simulink model "KalmanFilter_test"  (R2019a)
settings: Solver=FixedStepAuto  StartTime=0.0  StopTime=15  RelTol=1e-3  EnableMultiTasking=on
undefined symbols (not defined in the file): A, B, Ck, Discrete, Dk, i0, R, Time, Ts, u0, y0
libraries: MagnetoLibrary x3, ctrlSharedLib x1
settings Model: SimulationMode=external  ExtModeTrigDuration=2  Creator=jakub  LastModifiedBy=jakub
settings OptimizationCC: EnhancedBackFolding=on  PassReuseOutputArgsAs=Individual arguments  MaxStackSize=64  OptimizeBlockOrder=speed  DifferentSizesBufferReuse=on  OptimizationCustomize=off
settings DebuggingCC: ParameterTunabilityLossMsg=error
settings HardwareCC: ProdBitPerPointer=32  ProdBitPerSizeT=32  ProdBitPerPtrDiffT=32  ProdLargestAtomicInteger=Long  ProdLargestAtomicFloat=Double  ProdWordSize=32  ProdHWDeviceType=ARM Compatible->ARM Cortex
settings SFSimCC: MATLABDynamicMemAlloc=off
settings RTWCC: SystemTargetFile=ert.tlc  HardwareBoard=Arduino Due  TLCOptions=-aInlineSetEventsForThisBaseRateFcn=TLC_FALSE -aSuppressMultiTaskScheduler=TLC_FALSE -aRateBasedStepFcn=1  TemplateMakefile=ert_default_tmf  GenerateReport=on  Toolchain=Arduino ARM  BuildConfiguration=Faster Runs  IncludeHyperlinkInReport=on  LaunchReport=on  GenerateTraceInfo=on  GenerateTraceReport=on  GenerateTraceReportSl=on  GenerateTraceReportSf=on  GenerateTraceReportEml=on
settings CodeAppCC: ForceParamTrailComments=on  IgnoreCustomStorageClasses=off  OperatorAnnotations=on  SimulinkDataObjDesc=on  SFDataObjDesc=on  InsertBlockDesc=on
settings ERTTargetCC: SupportContinuousTime=on  SupportVariableSizeSignals=on  ExtModeStaticAllocSize=24576

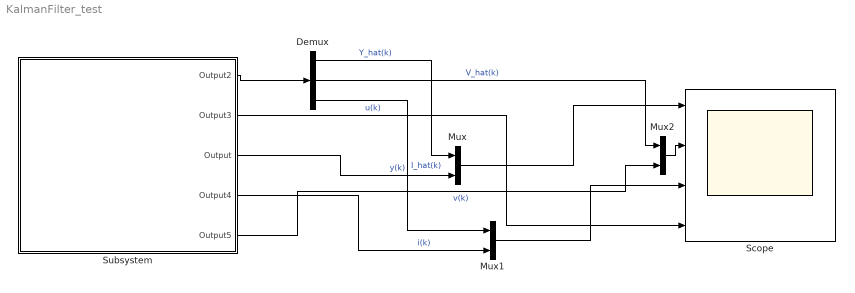
== system KalmanFilter_test ==
  Demux : Demux  Outputs=3
  Mux : Mux  Inputs=2
  Mux1 : Mux  Inputs=2
  Mux2 : Mux  Inputs=2
  Scope : Scope  NumInputPorts=4
  Subsystem : Subsystem
  wires:
  Subsystem/1(Output2) -> Demux/1
  Subsystem/3(Output) -> Mux/2  "y(k)"
  Subsystem/4(Output4) -> Mux1/2  "i(k)"
  Demux/3 -> Mux1/1  "I_hat(k)"
  Demux/1 -> Mux/1  "Y_hat(k)"
  Mux/1 -> Scope/1
  Demux/2 -> Mux2/1  "V_hat(k)"
  Mux1/1 -> Scope/3
  Subsystem/2(Output3) -> Scope/4  "u(k)"
  Subsystem/5(Output5) -> Mux2/2  "v(k)"
  Mux2/1 -> Scope/2

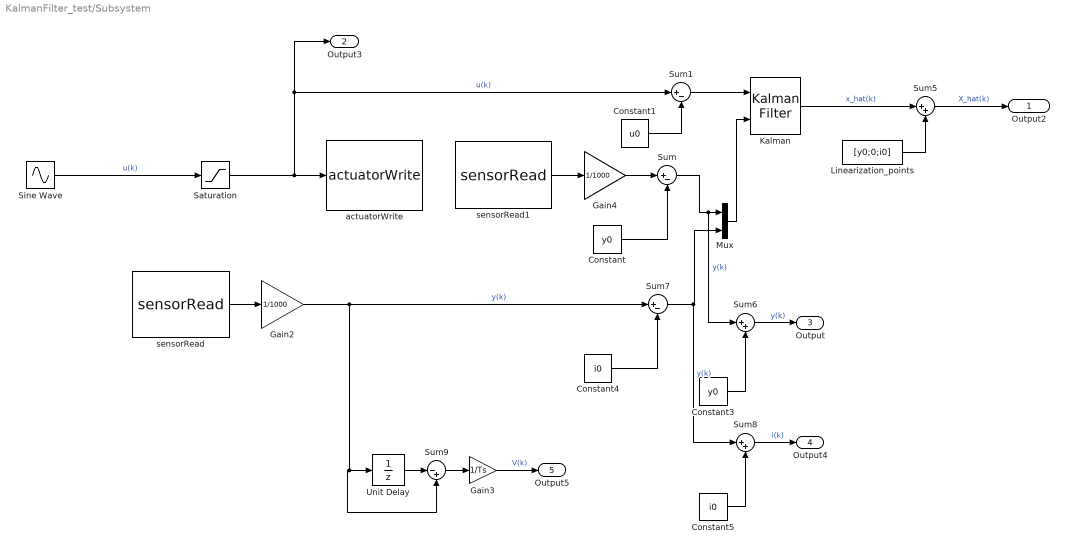
== system KalmanFilter_test/Subsystem ==
  Constant : Constant  Value=y0  SampleTime=Ts
  Constant1 : Constant  Value=u0  SampleTime=Ts
  Constant3 : Constant  Value=y0
  Constant4 : Constant  Value=i0
  Constant5 : Constant  Value=i0
  Gain2 : Gain  Gain=1/1000
  Gain3 : Gain  Gain=1/Ts
  Gain4 : Gain  Gain=1/1000
  Kalman : ctrlSharedLib/Kalman Filter  TimeDomain=Discrete-Time  UseCurrentEstimator=on  ModelSource=Individual A, B, C, D matrices  ModelSourceVariable=ss(0.95,1,1,0,1)  A=A  B=B  C=Ck  D=Dk  NumberOfStates=1  NumberOfInputs=1  NumberOfOutputs=1  InitialEstimateSource=Dialog  X0=[0.017-y0;0;0-i0]  P0=10  UseK=off  UseGH=off  NumberOfProcessNoiseInputs=1  G=1  TimeInvariantG=on  H=0  TimeInvariantH=on  Q=Q  TimeInvariantQ=on  R=R  TimeInvariantR=on  N=0  TimeInvariantN=on  AddInputPort=on  AddEnablePort=off  OutputEstimatedY=off  OutputP=off  Ts=Ts
  Linearization_points : Constant  Value=[y0;0;i0]
  Mux : Mux  Inputs=2
  Saturation : Saturate  UpperLimit=10  LowerLimit=0
  Sine Wave : Sin  Amplitude=5  Bias=5  Frequency=0.5  SampleTime=Ts
  Sum : Sum  Inputs=|+-
  Sum1 : Sum  Inputs=|+-
  Sum5 : Sum  Inputs=|++
  Sum6 : Sum  Inputs=|++
  Sum7 : Sum  Inputs=|+-
  Sum8 : Sum  Inputs=|++
  Sum9 : Sum  Inputs=|-+
  Unit Delay : UnitDelay  SampleTime=-1  HasFrameUpgradeWarning=on
  actuatorWrite : MagnetoLibrary/actuatorWrite  Board=DUE  Units=Volts
      settings: SourceProductName=AutomationShield
  sensorRead : MagnetoLibrary/sensorRead  board=DUE  sensor=Current [mA]  sampling=Ts
      settings: SourceProductName=AutomationShield
  sensorRead1 : MagnetoLibrary/sensorRead  board=DUE  sensor=Distance [mm]  sampling=Ts
      settings: SourceProductName=AutomationShield
  Output2 : Outport
  Output3 : Outport  Port=2
  Output : Outport  Port=3
  Output4 : Outport  Port=4
  Output5 : Outport  Port=5
  wires:
  Sum8/1 -> Output4/1  "i(k)"
  Mux/1 -> Kalman/2
  Sum7/1 -> Sum8/1, Mux/2  "y(k)"
  Sum5/1 -> Output2/1  "X_hat(k)"
  Constant4/1 -> Sum7/2
  Kalman/1 -> Sum5/1  "x_hat(k)"
  Sine Wave/1 -> Saturation/1  "u(k)"
  Constant/1 -> Sum/2
  Gain4/1 -> Sum/1
  Constant3/1 -> Sum6/2
  Sum6/1 -> Output/1  "y(k)"
  Constant5/1 -> Sum8/2
  Sum/1 -> Sum6/1, Mux/1  "y(k)"
  sensorRead1/1 -> Gain4/1
  Linearization_points/1 -> Sum5/2
  sensorRead/1 -> Gain2/1
  Saturation/1 -> actuatorWrite/1, Sum1/1, Output3/1  "u(k)"
  Constant1/1 -> Sum1/2
  Sum1/1 -> Kalman/1
  Gain3/1 -> Output5/1  "V(k)"
  Sum9/1 -> Gain3/1
  Gain2/1 -> Sum9/2, Unit Delay/1, Sum7/1  "y(k)"
  Unit Delay/1 -> Sum9/1
